simulink library "actuators_lib_torques"  (R2018b)
settings: Solver=VariableStepAuto  StartTime=0.0  StopTime=10.0  RelTol=1e-3
libraries: mtq_lib x1, rwa_assembly_torqueinput_lib x1
settings Model: Creator=colem  LastModifiedBy=colem

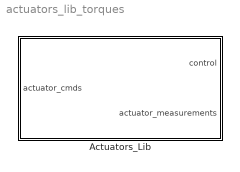
== system actuators_lib_torques ==
  Actuators_Lib : Subsystem

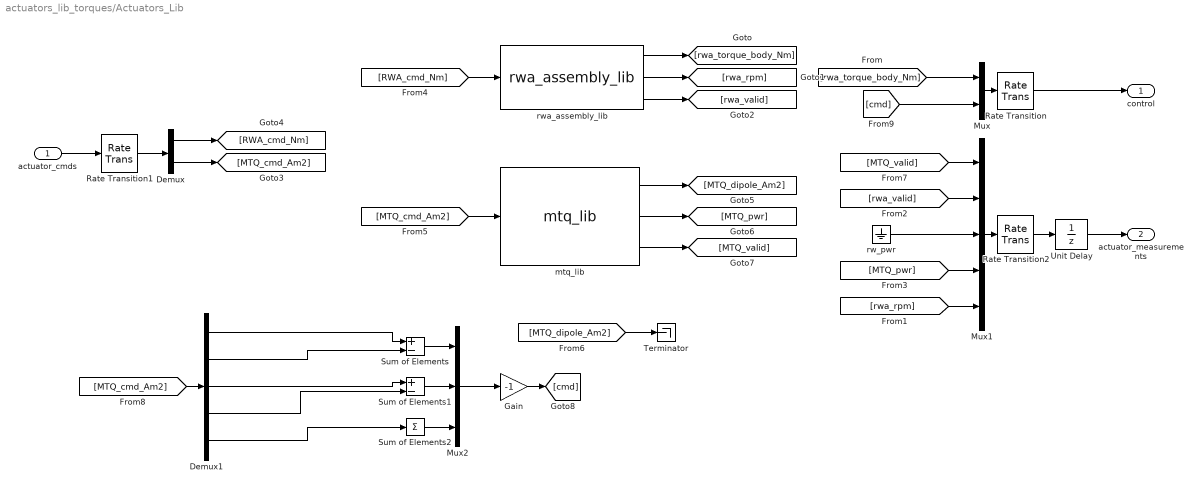
== system actuators_lib_torques/Actuators_Lib ==
  actuator_cmds : Inport
  Demux : Demux  Outputs=[4 5]
  Demux1 : Demux  Outputs=5
  Gain : Gain  Gain=-1
  Mux : Mux  Inputs=[3 3]
  Mux1 : Mux  Inputs=[5 4 1 1 4]
  Mux2 : Mux  Inputs=3
  Rate Transition : RateTransition
  Rate Transition1 : RateTransition  OutPortSampleTime=simParams.actuators.sample_time_s
  Rate Transition2 : RateTransition
  Sum of Elements : Sum  Inputs=+-
  Sum of Elements1 : Sum  Inputs=+-
  Sum of Elements2 : Sum  Inputs=+
  Terminator : Terminator
  Unit Delay : UnitDelay  SampleTime=-1
  mtq_lib : mtq_lib/mtq_lib  SystemSampleTime=-1
  rw_pwr : Ground
  rwa_assembly_lib : rwa_assembly_torqueinput_lib/rwa_assembly_lib  SystemSampleTime=-1
  control : Outport
  actuator_measurements : Outport  Port=2
  wires:
  Rate Transition/1 -> control/1
  actuator_cmds/1 -> Rate Transition1/1
  rwa_assembly_lib/2 -> [rwa_rpm]
  rwa_assembly_lib/3 -> [rwa_valid]
  rwa_assembly_lib/1 -> [rwa_torque_body_Nm]
  [rwa_rpm] -> Mux1/5
  [rwa_valid] -> Mux1/2
  Mux1/1 -> Rate Transition2/1
  Rate Transition1/1 -> Demux/1
  [MTQ_dipole_Am2] -> Terminator/1
  [rwa_torque_body_Nm] -> Mux/1
  Mux/1 -> Rate Transition/1
  Demux/2 -> [MTQ_cmd_Am2]
  Demux/1 -> [RWA_cmd_Nm]
  [RWA_cmd_Nm] -> rwa_assembly_lib/1
  [MTQ_cmd_Am2] -> mtq_lib/1
  mtq_lib/2 -> [MTQ_pwr]
  mtq_lib/1 -> [MTQ_dipole_Am2]
  mtq_lib/3 -> [MTQ_valid]
  [MTQ_pwr] -> Mux1/4
  rw_pwr/1 -> Mux1/3
  [MTQ_valid] -> Mux1/1
  Sum of Elements1/1 -> Mux2/2
  Demux1/3 -> Sum of Elements1/1
  Demux1/5 -> Sum of Elements2/1
  Sum of Elements2/1 -> Mux2/3
  Demux1/1 -> Sum of Elements/1
  Mux2/1 -> Gain/1
  Sum of Elements/1 -> Mux2/1
  [cmd] -> Mux/2
  Gain/1 -> [cmd]
  [MTQ_cmd_Am2] -> Demux1/1
  Demux1/2 -> Sum of Elements/2
  Demux1/4 -> Sum of Elements1/2
  Rate Transition2/1 -> Unit Delay/1
  Unit Delay/1 -> actuator_measurements/1
